simulink model "Ex4"  (R2017a)
settings: Solver=ode45  StartTime=0.0  StopTime=10.0  RelTol=1e-3  EnableMultiTasking=on
libraries: simulink x1
settings Model: Creator=99641  LastModifiedBy=99641
settings DataIOCC: LimitDataPoints=on  SaveFormat=Array
settings OptimizationCC: LifeSpan=inf
settings DebuggingCC: SolverPrmCheckMsg=warning  SFUnexpectedBacktrackingDiag=warning  SFNoUnconditionalDefaultTransitionDiag=warning  SFExecutionAtInitializationDiag=none
settings HardwareCC: ProdBitPerPointer=32  ProdBitPerSizeT=32  ProdBitPerPtrDiffT=32  ProdLargestAtomicFloat=None  ProdIntDivRoundTo=Undefined  ProdEndianess=Unspecified  ProdWordSize=32  ProdHWDeviceType=32-bit Generic
settings ModelReferenceCC: PropagateSignalLabelsOutOfModel=off
settings GRTTargetCC: TargetLangStandard=C89/C90 (ANSI)  GeneratePreprocessorConditionals=Disable all
settings ConfigComp: CovMetricSettings=dw  CovHtmlReporting=on  CovSaveCumulativeToWorkspaceVar=on  CovSaveSingleToWorkspaceVar=on  CovExternalEMLEnable=off  CovSFcnEnable=off

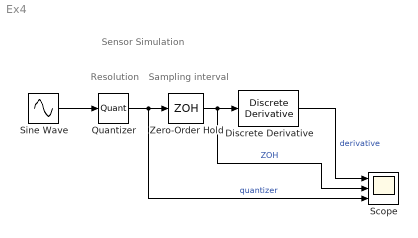
== system Ex4 ==
  note: Sampling interval
  note: Resolution
  note: Sensor Simulation
  Discrete Derivative : simulink/Discrete/Discrete Derivative  gainval=1.0  ICPrevScaledInput=0.0  InputProcessing=Inherited  OutMin=[]  OutMax=[]  OutDataType=fixdt(1, 16)  OutScaling=2^-10  DoSatur=off
  Quantizer : Quantizer  QuantizationInterval=2*pi/8192
  Scope : Scope  NumInputPorts=3
  Sine Wave : Sin  SampleTime=0
  Zero-Order Hold : ZeroOrderHold  SampleTime=0.01
  wires:
  Sine Wave/1 -> Quantizer/1
  Zero-Order Hold/1 -> Scope/2, Discrete Derivative/1  "ZOH"
  Quantizer/1 -> Scope/3, Zero-Order Hold/1  "quantizer"
  Discrete Derivative/1 -> Scope/1  "derivative"
